simulink model "iiwa_v_1"  (R2015a)
settings: Solver=ode3  StartTime=0.0  StopTime=10  FixedStep=0.001  RelTol=1e-3
undefined symbols (not defined in the file or in its folder): X, Y, Z
libraries: sm_lib x40, nesl_utility x22
settings Model: Creator=alaa.alassi1  LastModifiedBy=robotic

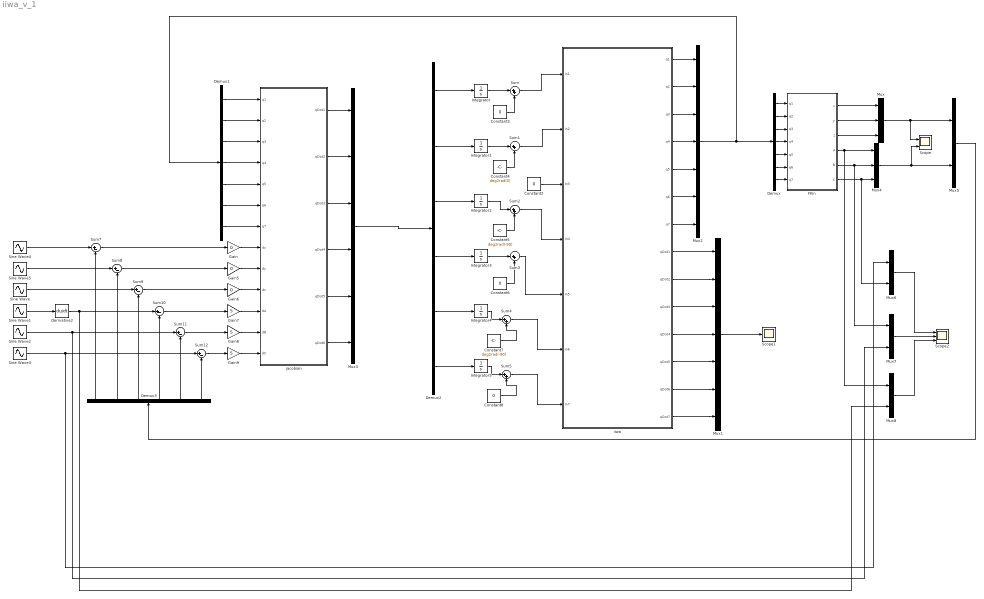
== system iiwa_v_1 ==
  Constant{2..3,6,8} (4 alike) : Constant  Value=0
  Constant4 : Constant  Value=deg2rad(0)
  Constant5 : Constant  Value=deg2rad(-90)
  Constant7 : Constant  Value=deg2rad(-90)
  Demux : Demux  Outputs=7
  Demux1 : Demux  Outputs=7
  Demux2 : Demux  Outputs=6
  Demux3 : Demux  Outputs=6
  Derivative2 : Derivative
  FKin : MATLAB Function  TreatAsAtomicUnit=on
  Gain : Gain  Gain=0
  Gain5 : Gain  Gain=0
  Gain6 : Gain  Gain=0
  Gain7 : Gain  Gain=5
  Gain8 : Gain  Gain=5
  Gain9 : Gain  Gain=5
  Integrator{,1..5} (6 alike) : Integrator
  Mux : Mux  Inputs=3
  Mux1 : Mux  Inputs=7
  Mux2 : Mux  Inputs=7
  Mux3 : Mux  Inputs=6
  Mux4 : Mux  Inputs=3
  Mux{5..8} (4 alike) : Mux  Inputs=2
  Scope : Scope  NumInputPorts=2
      settings: YMin=-5~-5  YMax=5~5
  Scope1 : Scope
  Scope2 : Scope  NumInputPorts=3
      settings: YMin=-5~-5~-5  YMax=5~5~5  SaveName=ScopeData2
  Sine Wave : Sin  Amplitude=0.1  Bias=0.7067  Frequency=4  SampleTime=0
  Sine Wave1 : Sin  SampleTime=0
  Sine Wave2 : Sin  SampleTime=0
  Sine Wave3 : Sin  SampleTime=0
  Sine Wave4 : Sin  Amplitude=0.1  Bias=0.7067  Frequency=4  SampleTime=0
  Sine Wave5 : Sin  Amplitude=0.1  Bias=0.7067  Frequency=4  SampleTime=0
  Sum{,1..5} (6 alike) : Sum  Inputs=|++
  Sum{7..12} (6 alike) : Sum  Inputs=|+-
  iiwa : Subsystem
  jacobian : MATLAB Function  TreatAsAtomicUnit=on
  wires:
  FKin/1(x) -> Mux/1
  FKin/2(y) -> Mux/2
  FKin/3(z) -> Mux/3
  Mux/1 -> Scope/1, Mux5/1
  Mux1/1 -> Scope1/1
  iiwa/8(qDot1) -> Mux1/1
  iiwa/9(qDot2) -> Mux1/2
  iiwa/10(qDot3) -> Mux1/3
  iiwa/11(qDot4) -> Mux1/4
  iiwa/12(qDot5) -> Mux1/5
  iiwa/13(qDot6) -> Mux1/6
  iiwa/14(qDot7) -> Mux1/7
  iiwa/1(q1) -> Mux2/1
  iiwa/3(q3) -> Mux2/3
  iiwa/4(q4) -> Mux2/4
  iiwa/5(q5) -> Mux2/5
  iiwa/6(q6) -> Mux2/6
  iiwa/7(q7) -> Mux2/7
  Demux/1 -> FKin/1(q1)
  Demux/2 -> FKin/2(q2)
  Demux/3 -> FKin/3(q3)
  Demux/4 -> FKin/4(q4)
  Demux/5 -> FKin/5(q5)
  Demux/6 -> FKin/6(q6)
  Demux/7 -> FKin/7(q7)
  Demux1/1 -> jacobian/1(q1)
  Demux1/2 -> jacobian/2(q2)
  Demux1/3 -> jacobian/3(q3)
  Demux1/4 -> jacobian/4(q4)
  Demux1/5 -> jacobian/5(q5)
  Demux1/6 -> jacobian/6(q6)
  Demux1/7 -> jacobian/7(q7)
  Mux2/1 -> Demux1/1, Demux/1
  jacobian/1(qDot1) -> Mux3/1
  jacobian/2(qDot2) -> Mux3/2
  jacobian/3(qDot3) -> Mux3/3
  jacobian/4(qDot4) -> Mux3/4
  jacobian/5(qDot5) -> Mux3/5
  jacobian/6(qDot6) -> Mux3/6
  Constant2/1 -> iiwa/3(In3)
  Demux2/1 -> Integrator/1
  Demux2/2 -> Integrator1/1
  Demux2/3 -> Integrator2/1
  Demux2/4 -> Integrator3/1
  Demux2/5 -> Integrator4/1
  Demux2/6 -> Integrator5/1
  Integrator/1 -> Sum/1
  Sum/1 -> iiwa/1(In1)
  Constant3/1 -> Sum/2
  Integrator1/1 -> Sum1/1
  Sum1/1 -> iiwa/2(In2)
  Constant4/1 -> Sum1/2
  Integrator2/1 -> Sum2/1
  Sum2/1 -> iiwa/4(In4)
  Constant5/1 -> Sum2/2
  Integrator3/1 -> Sum3/1
  Sum3/1 -> iiwa/5(In5)
  Constant6/1 -> Sum3/2
  Integrator4/1 -> Sum4/1
  Sum4/1 -> iiwa/6(In6)
  Constant7/1 -> Sum4/2
  Integrator5/1 -> Sum5/1
  Sum5/1 -> iiwa/7(In7)
  Constant8/1 -> Sum5/2
  Mux3/1 -> Demux2/1
  iiwa/2(q2) -> Mux2/2
  FKin/4(A) -> Mux8/1, Mux4/1
  FKin/5(B) -> Mux7/1, Mux4/2
  FKin/6(C) -> Mux6/2, Mux4/3
  Mux4/1 -> Scope/2, Mux5/2
  Gain/1 -> jacobian/8(dx)
  Gain5/1 -> jacobian/9(dy)
  Gain6/1 -> jacobian/10(dz)
  Gain7/1 -> jacobian/11(dA)
  Gain8/1 -> jacobian/12(dB)
  Gain9/1 -> jacobian/13(dC)
  Sum7/1 -> Gain/1
  Sum8/1 -> Gain5/1
  Sum9/1 -> Gain6/1
  Sum10/1 -> Gain7/1
  Sum11/1 -> Gain8/1
  Sum12/1 -> Gain9/1
  Mux5/1 -> Demux3/1
  Demux3/6 -> Sum12/2
  Demux3/1 -> Sum7/2
  Demux3/2 -> Sum8/2
  Demux3/3 -> Sum9/2
  Demux3/4 -> Sum10/2
  Demux3/5 -> Sum11/2
  Sine Wave/1 -> Sum9/1
  Sine Wave4/1 -> Sum7/1
  Sine Wave5/1 -> Sum8/1
  Mux6/1 -> Scope2/1
  Sine Wave2/1 -> Mux7/2, Sum11/1
  Sine Wave1/1 -> Derivative2/1
  Mux7/1 -> Scope2/2
  Mux8/1 -> Scope2/3
  Derivative2/1 -> Sum10/1, Mux8/2
  Sine Wave3/1 -> Sum12/1, Mux6/1

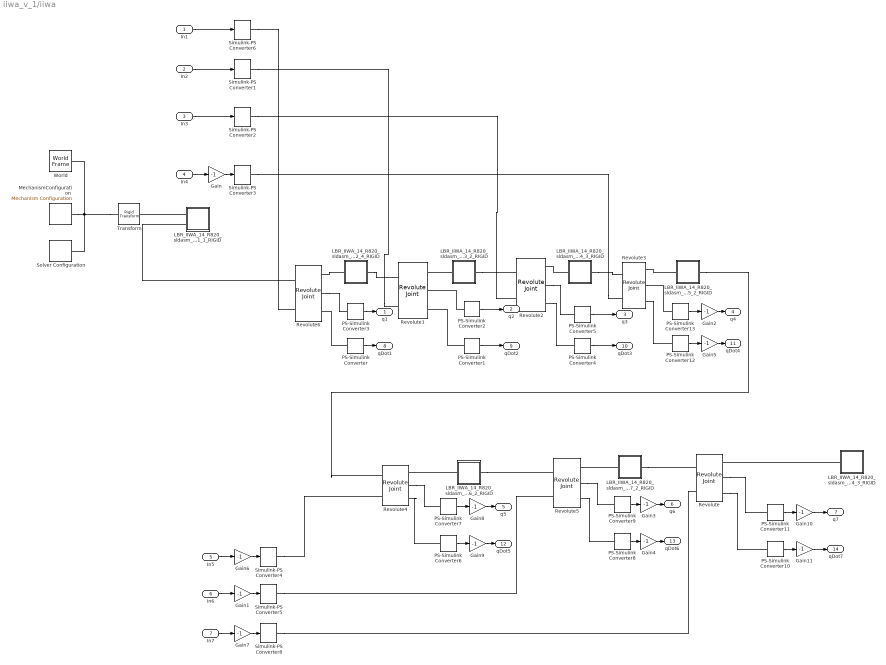
== system iiwa_v_1/iiwa ==
  In1 : Inport
  In2 : Inport  Port=2
  In3 : Inport  Port=3
  In4 : Inport  Port=4
  In5 : Inport  Port=5
  In6 : Inport  Port=6
  In7 : Inport  Port=7
  Gain{,1..11} (12 alike) : Gain  Gain=-1
  LBR_IIWA_14_R820_sldasm_Part_14_3_RIGID : Subsystem
  LBR_IIWA_14_R820_sldasm_Part_1_1_RIGID : Subsystem
  LBR_IIWA_14_R820_sldasm_Part_2_4_RIGID : Subsystem
  LBR_IIWA_14_R820_sldasm_Part_3_2_RIGID : Subsystem
  LBR_IIWA_14_R820_sldasm_Part_4_3_RIGID : Subsystem
  LBR_IIWA_14_R820_sldasm_Part_5_2_RIGID : Subsystem
  LBR_IIWA_14_R820_sldasm_Part_6_2_RIGID : Subsystem
  LBR_IIWA_14_R820_sldasm_Part_7_2_RIGID : Subsystem
  MechanismConfiguration : sm_lib/Utilities/Mechanism Configuration  UniformGravity=Constant  GravityVector=[0 -0 -0]  GravityUnits=m/s^2  LinearizationDelta=0.001  BlockFunction=simmechanics.library.utilities.mechanism_configuration
  PS-Simulink Converter{,1..13} (14 alike) : nesl_utility/PS-Simulink Converter  PhysicalDomain=network_engine_domain  SubClassName=ps_output  LeftPortType=input  RightPortType=output  PseudoPeriodic=off  Frequencies=[]  Unit=1  AffineConversion=off
  Revolute : sm_lib/Joints/Revolute Joint  SenseConstraintForce=off  SenseConstraintForceX=off  SenseConstraintForceY=off  SenseConstraintForceZ=off  SenseConstraintTorque=off  SenseConstraintTorqueX=off  SenseConstraintTorqueY=off  SenseConstraintTorqueZ=off  SenseTotalForce=off  SenseTotalForceX=off  SenseTotalForceY=off  SenseTotalForceZ=off  SenseTotalTorque=off  SenseTotalTorqueX=off  SenseTotalTorqueY=off  SenseTotalTorqueZ=off  CompositeWrenchDir=FollowerOnBase  CompositeWrenchFrame=BaseFrame  EquilibriumPosition=0  EquilibriumPositionUnits=rad  SpringStiffness=0  SpringStiffnessUnits=m*N/rad  DampingCoefficient=0  DampingCoefficientUnits=m*s*N/rad  TorqueActuationMode=ComputedTorque  MotionActuationMode=InputMotion  SensePosition=on  SenseVelocity=on  SenseAcceleration=off  SenseTorqueForce=off  PositionTargetSpecify=off  PositionTargetPriority=Low  PositionTargetValue=0  PositionTargetValueUnits=deg  VelocityTargetSpecify=off  VelocityTargetPriority=High  VelocityTargetValue=0  VelocityTargetValueUnits=deg/s  BlockFunction=simmechanics.library.joints.revolute_joint
  Revolute1 : sm_lib/Joints/Revolute Joint  SenseConstraintForce=off  SenseConstraintForceX=off  SenseConstraintForceY=off  SenseConstraintForceZ=off  SenseConstraintTorque=off  SenseConstraintTorqueX=off  SenseConstraintTorqueY=off  SenseConstraintTorqueZ=off  SenseTotalForce=off  SenseTotalForceX=off  SenseTotalForceY=off  SenseTotalForceZ=off  SenseTotalTorque=off  SenseTotalTorqueX=off  SenseTotalTorqueY=off  SenseTotalTorqueZ=off  CompositeWrenchDir=FollowerOnBase  CompositeWrenchFrame=BaseFrame  EquilibriumPosition=0  EquilibriumPositionUnits=rad  SpringStiffness=0  SpringStiffnessUnits=m*N/rad  DampingCoefficient=0  DampingCoefficientUnits=m*s*N/rad  TorqueActuationMode=ComputedTorque  MotionActuationMode=InputMotion  SensePosition=on  SenseVelocity=on  SenseAcceleration=off  SenseTorqueForce=off  PositionTargetSpecify=on  PositionTargetPriority=Low  PositionTargetValue=0  PositionTargetValueUnits=deg  VelocityTargetSpecify=off  VelocityTargetPriority=Low  VelocityTargetValue=0  VelocityTargetValueUnits=deg/s  BlockFunction=simmechanics.library.joints.revolute_joint
  Revolute2 : sm_lib/Joints/Revolute Joint  SenseConstraintForce=off  SenseConstraintForceX=off  SenseConstraintForceY=off  SenseConstraintForceZ=off  SenseConstraintTorque=off  SenseConstraintTorqueX=off  SenseConstraintTorqueY=off  SenseConstraintTorqueZ=off  SenseTotalForce=off  SenseTotalForceX=off  SenseTotalForceY=off  SenseTotalForceZ=off  SenseTotalTorque=off  SenseTotalTorqueX=off  SenseTotalTorqueY=off  SenseTotalTorqueZ=off  CompositeWrenchDir=FollowerOnBase  CompositeWrenchFrame=BaseFrame  EquilibriumPosition=0  EquilibriumPositionUnits=rad  SpringStiffness=0  SpringStiffnessUnits=m*N/rad  DampingCoefficient=0  DampingCoefficientUnits=m*s*N/rad  TorqueActuationMode=ComputedTorque  MotionActuationMode=InputMotion  SensePosition=on  SenseVelocity=on  SenseAcceleration=off  SenseTorqueForce=off  PositionTargetSpecify=off  PositionTargetPriority=Low  PositionTargetValue=0  PositionTargetValueUnits=deg  VelocityTargetSpecify=off  VelocityTargetPriority=High  VelocityTargetValue=0  VelocityTargetValueUnits=deg/s  BlockFunction=simmechanics.library.joints.revolute_joint
  Revolute3 : sm_lib/Joints/Revolute Joint  SenseConstraintForce=off  SenseConstraintForceX=off  SenseConstraintForceY=off  SenseConstraintForceZ=off  SenseConstraintTorque=off  SenseConstraintTorqueX=off  SenseConstraintTorqueY=off  SenseConstraintTorqueZ=off  SenseTotalForce=off  SenseTotalForceX=off  SenseTotalForceY=off  SenseTotalForceZ=off  SenseTotalTorque=off  SenseTotalTorqueX=off  SenseTotalTorqueY=off  SenseTotalTorqueZ=off  CompositeWrenchDir=FollowerOnBase  CompositeWrenchFrame=BaseFrame  EquilibriumPosition=0  EquilibriumPositionUnits=rad  SpringStiffness=0  SpringStiffnessUnits=m*N/rad  DampingCoefficient=0  DampingCoefficientUnits=m*s*N/rad  TorqueActuationMode=ComputedTorque  MotionActuationMode=InputMotion  SensePosition=on  SenseVelocity=on  SenseAcceleration=off  SenseTorqueForce=off  PositionTargetSpecify=off  PositionTargetPriority=Low  PositionTargetValue=60  PositionTargetValueUnits=deg  VelocityTargetSpecify=off  VelocityTargetPriority=High  VelocityTargetValue=0  VelocityTargetValueUnits=deg/s  BlockFunction=simmechanics.library.joints.revolute_joint
  Revolute4 : sm_lib/Joints/Revolute Joint  SenseConstraintForce=off  SenseConstraintForceX=off  SenseConstraintForceY=off  SenseConstraintForceZ=off  SenseConstraintTorque=off  SenseConstraintTorqueX=off  SenseConstraintTorqueY=off  SenseConstraintTorqueZ=off  SenseTotalForce=off  SenseTotalForceX=off  SenseTotalForceY=off  SenseTotalForceZ=off  SenseTotalTorque=off  SenseTotalTorqueX=off  SenseTotalTorqueY=off  SenseTotalTorqueZ=off  CompositeWrenchDir=FollowerOnBase  CompositeWrenchFrame=BaseFrame  EquilibriumPosition=0  EquilibriumPositionUnits=rad  SpringStiffness=0  SpringStiffnessUnits=m*N/rad  DampingCoefficient=0  DampingCoefficientUnits=m*s*N/rad  TorqueActuationMode=ComputedTorque  MotionActuationMode=InputMotion  SensePosition=on  SenseVelocity=on  SenseAcceleration=off  SenseTorqueForce=off  PositionTargetSpecify=off  PositionTargetPriority=Low  PositionTargetValue=0  PositionTargetValueUnits=deg  VelocityTargetSpecify=off  VelocityTargetPriority=High  VelocityTargetValue=0  VelocityTargetValueUnits=deg/s  BlockFunction=simmechanics.library.joints.revolute_joint
  Revolute5 : sm_lib/Joints/Revolute Joint  SenseConstraintForce=off  SenseConstraintForceX=off  SenseConstraintForceY=off  SenseConstraintForceZ=off  SenseConstraintTorque=off  SenseConstraintTorqueX=off  SenseConstraintTorqueY=off  SenseConstraintTorqueZ=off  SenseTotalForce=off  SenseTotalForceX=off  SenseTotalForceY=off  SenseTotalForceZ=off  SenseTotalTorque=off  SenseTotalTorqueX=off  SenseTotalTorqueY=off  SenseTotalTorqueZ=off  CompositeWrenchDir=FollowerOnBase  CompositeWrenchFrame=BaseFrame  EquilibriumPosition=0  EquilibriumPositionUnits=rad  SpringStiffness=0  SpringStiffnessUnits=m*N/rad  DampingCoefficient=0  DampingCoefficientUnits=m*s*N/rad  TorqueActuationMode=ComputedTorque  MotionActuationMode=InputMotion  SensePosition=on  SenseVelocity=on  SenseAcceleration=off  SenseTorqueForce=off  PositionTargetSpecify=off  PositionTargetPriority=Low  PositionTargetValue=-90  PositionTargetValueUnits=deg  VelocityTargetSpecify=off  VelocityTargetPriority=High  VelocityTargetValue=0  VelocityTargetValueUnits=deg/s  BlockFunction=simmechanics.library.joints.revolute_joint
  Revolute6 : sm_lib/Joints/Revolute Joint  SenseConstraintForce=off  SenseConstraintForceX=off  SenseConstraintForceY=off  SenseConstraintForceZ=off  SenseConstraintTorque=off  SenseConstraintTorqueX=off  SenseConstraintTorqueY=off  SenseConstraintTorqueZ=off  SenseTotalForce=off  SenseTotalForceX=off  SenseTotalForceY=off  SenseTotalForceZ=off  SenseTotalTorque=off  SenseTotalTorqueX=off  SenseTotalTorqueY=off  SenseTotalTorqueZ=off  CompositeWrenchDir=FollowerOnBase  CompositeWrenchFrame=BaseFrame  EquilibriumPosition=0  EquilibriumPositionUnits=rad  SpringStiffness=0  SpringStiffnessUnits=m*N/rad  DampingCoefficient=0  DampingCoefficientUnits=m*s*N/rad  TorqueActuationMode=ComputedTorque  MotionActuationMode=InputMotion  SensePosition=on  SenseVelocity=on  SenseAcceleration=off  SenseTorqueForce=off  PositionTargetSpecify=off  PositionTargetPriority=Low  PositionTargetValue=0  PositionTargetValueUnits=deg  VelocityTargetSpecify=off  VelocityTargetPriority=High  VelocityTargetValue=1  VelocityTargetValueUnits=rad/s  BlockFunction=simmechanics.library.joints.revolute_joint
  Simulink-PS Converter{1..5,8} (6 alike) : nesl_utility/Simulink-PS Converter  PhysicalDomain=network_engine_domain  SubClassName=ps_input  LeftPortType=input  RightPortType=output  PseudoPeriodic=off  Frequencies=[]  NoiseDistribution=none  NoiseParameters=[]  Unit=rad  AffineConversion=on  InputFiltering=on  SimscapeFilterOrder=2  InputFilterTimeConstant=0.001  UdotUserProvided=1
  Simulink-PS Converter6 : nesl_utility/Simulink-PS Converter  PhysicalDomain=network_engine_domain  SubClassName=ps_input  LeftPortType=input  RightPortType=output  PseudoPeriodic=off  Frequencies=[]  NoiseDistribution=none  NoiseParameters=[]  Unit=rad  AffineConversion=on  InputFiltering=on  SimscapeFilterOrder=2  InputFilterTimeConstant=0.001  UdotUserProvided=2
  Solver Configuration : nesl_utility/Solver Configuration  PhysicalDomain=network_engine_domain  SubClassName=solver  LeftPortType=input  RightPortType=generic  Accelerate=off  Tones=[]  Harmonics=[]  SimulateNoise=off  Profile=off  UseLocalSampling=off  EnableSwitchedLinearOptims=on  FrequencyDomain=off  UseCCode=off  RelTol=0.001  AbsTol=1e-06  MinStep=1e-09  ToWorkspace=off  RevertToSquareIcSolve=off  NumHomotopyIterations=100  DoDC=off  ResidualTolerance=1e-09  UseLocalSolver=off  LocalSolverChoice=NE_BACKWARD_EULER_ADVANCER  LocalSolverSampleTime=0.001  DoFixedCost=off  MaxNonlinIter=3  MaxModeIter=2  LinearAlgebra=Sparse  DelaysMemoryBudget=1024  AutomaticFiltering=on  FilteringTimeConstant=0.001
  Transform : sm_lib/Frames and Transforms/Rigid Transform  TranslationMethod=Cartesian  TranslationLengthUnit=mm  TranslationStandardAxis=+Z  TranslationStandardOffset=0  TranslationCartesianOffset=[119.17615287075404 -10.082715490568717 -56.037583436526596]  TranslationROffset=0  TranslationROffsetUnits=m  TranslationZOffset=0  TranslationZOffsetUnits=m  TranslationThetaOffset=0  TranslationThetaOffsetUnits=deg  RotationMethod=None  RotationAngleUnits=deg  RotationStandardAxis=+Z  RotationAngle=0.0  RotationArbitraryAxis=[0 0 1]  FollAlignAxisA=+X  BaseAlignAxisA=+Y  FollAlignAxisB=+Y  BaseAlignAxisB=+Z  RotationMatrix=[1 0 0; 0 1 0; 0 0 1]  BlockFunction=simmechanics.library.frames_transforms.rigid_transform
  World : sm_lib/Frames and Transforms/World Frame  BlockFunction=simmechanics.library.frames_transforms.world_frame
  q1 : Outport
  q2 : Outport  Port=2
  q3 : Outport  Port=3
  q4 : Outport  Port=4
  q5 : Outport  Port=5
  q6 : Outport  Port=6
  q7 : Outport  Port=7
  qDot1 : Outport  Port=8
  qDot2 : Outport  Port=9
  qDot3 : Outport  Port=10
  qDot4 : Outport  Port=11
  qDot5 : Outport  Port=12
  qDot6 : Outport  Port=13
  qDot7 : Outport  Port=14
  wires:
  PS-Simulink Converter12/1 -> Gain5/1
  PS-Simulink Converter13/1 -> Gain2/1
  In3/1 -> Simulink-PS Converter2/1
  In6/1 -> Gain1/1
  PS-Simulink Converter11/1 -> Gain10/1
  In1/1 -> Simulink-PS Converter6/1
  In2/1 -> Simulink-PS Converter1/1
  PS-Simulink Converter5/1 -> q3/1
  PS-Simulink Converter1/1 -> qDot2/1
  PS-Simulink Converter4/1 -> qDot3/1
  PS-Simulink Converter6/1 -> Gain9/1
  PS-Simulink Converter2/1 -> q2/1
  PS-Simulink Converter3/1 -> q1/1
  PS-Simulink Converter/1 -> qDot1/1
  Gain/1 -> Simulink-PS Converter3/1
  In4/1 -> Gain/1
  Gain1/1 -> Simulink-PS Converter5/1
  Gain2/1 -> q4/1
  PS-Simulink Converter9/1 -> Gain3/1
  Gain3/1 -> q6/1
  PS-Simulink Converter8/1 -> Gain4/1
  Gain4/1 -> qDot6/1
  Gain5/1 -> qDot4/1
  In5/1 -> Gain6/1
  Gain6/1 -> Simulink-PS Converter4/1
  Gain7/1 -> Simulink-PS Converter8/1
  In7/1 -> Gain7/1
  PS-Simulink Converter7/1 -> Gain8/1
  Gain8/1 -> q5/1
  Gain9/1 -> qDot5/1
  Gain10/1 -> q7/1
  PS-Simulink Converter10/1 -> Gain11/1
  Gain11/1 -> qDot7/1
  connections:
  LBR_IIWA_14_R820_sldasm_Part_2_4_RIGID/RConn1 -- Revolute1/LConn1
  LBR_IIWA_14_R820_sldasm_Part_14_3_RIGID/LConn1 -- Revolute/RConn1
  LBR_IIWA_14_R820_sldasm_Part_3_2_RIGID/RConn1 -- Revolute2/LConn1
  LBR_IIWA_14_R820_sldasm_Part_4_3_RIGID/LConn1 -- Revolute2/RConn1
  LBR_IIWA_14_R820_sldasm_Part_3_2_RIGID/LConn1 -- Revolute1/RConn1
  Transform/LConn1 -- World/RConn1 -- Solver Configuration/RConn1 -- MechanismConfiguration/RConn1
  LBR_IIWA_14_R820_sldasm_Part_6_2_RIGID/RConn1 -- Revolute5/LConn1
  LBR_IIWA_14_R820_sldasm_Part_5_2_RIGID/RConn1 -- Revolute4/LConn1
  LBR_IIWA_14_R820_sldasm_Part_7_2_RIGID/LConn1 -- Revolute5/RConn1
  LBR_IIWA_14_R820_sldasm_Part_1_1_RIGID/LConn1 -- Transform/RConn1
  LBR_IIWA_14_R820_sldasm_Part_7_2_RIGID/RConn1 -- Revolute/LConn1
  LBR_IIWA_14_R820_sldasm_Part_6_2_RIGID/LConn1 -- Revolute4/RConn1
  Revolute3/RConn3 -- PS-Simulink Converter12/LConn1
  PS-Simulink Converter1/LConn1 -- Revolute1/RConn3
  PS-Simulink Converter13/LConn1 -- Revolute3/RConn2
  PS-Simulink Converter/LConn1 -- Revolute6/RConn3
  Revolute6/RConn2 -- PS-Simulink Converter3/LConn1
  Simulink-PS Converter1/RConn1 -- Revolute1/LConn2
  LBR_IIWA_14_R820_sldasm_Part_4_3_RIGID/RConn1 -- Revolute3/LConn1
  LBR_IIWA_14_R820_sldasm_Part_5_2_RIGID/LConn1 -- Revolute3/RConn1
  LBR_IIWA_14_R820_sldasm_Part_1_1_RIGID/LConn2 -- Revolute6/LConn1
  Revolute6/RConn1 -- LBR_IIWA_14_R820_sldasm_Part_2_4_RIGID/LConn1
  Simulink-PS Converter2/RConn1 -- Revolute2/LConn2
  Simulink-PS Converter3/RConn1 -- Revolute3/LConn2
  Simulink-PS Converter4/RConn1 -- Revolute4/LConn2
  Simulink-PS Converter5/RConn1 -- Revolute5/LConn2
  Simulink-PS Converter8/RConn1 -- Revolute/LConn2
  Revolute/RConn2 -- PS-Simulink Converter11/LConn1
  PS-Simulink Converter2/LConn1 -- Revolute1/RConn2
  Revolute/RConn3 -- PS-Simulink Converter10/LConn1
  Simulink-PS Converter6/RConn1 -- Revolute6/LConn2
  Revolute2/RConn3 -- PS-Simulink Converter4/LConn1
  Revolute4/RConn2 -- PS-Simulink Converter7/LConn1
  Revolute5/RConn3 -- PS-Simulink Converter8/LConn1
  Revolute2/RConn2 -- PS-Simulink Converter5/LConn1
  Revolute4/RConn3 -- PS-Simulink Converter6/LConn1
  Revolute5/RConn2 -- PS-Simulink Converter9/LConn1

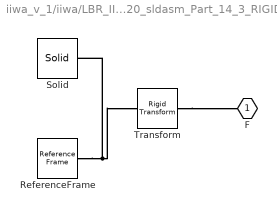
== system iiwa_v_1/iiwa/LBR_IIWA_14_R820_sldasm_Part_14_3_RIGID ==
  ReferenceFrame : sm_lib/Frames and Transforms/Reference Frame  BlockFunction=simmechanics.library.frames_transforms.reference_frame
  Solid : sm_lib/Body Elements/Solid  InertiaType=Custom  Mass=0.31121894529121702  MassUnits=kg  CenterOfMass=[0.014528621653147699 0.087032798846967588 1278.3655137735861]  CenterOfMassUnits=mm  MomentsOfInertia=[222.42389382502736 221.16881041551065 342.04081748406088]  MomentsOfInertiaUnits=kg*mm^2  ProductsOfInertia=[-0.22311621312267468 -0.062033496808603497 0.11472620552029689]  ProductsOfInertiaUnits=kg*mm^2  DensityBased=on  Density=1000  DensityUnits=kg/(m^3)  GraphicType=FromGeometry  MarkerShape=Sphere  MarkerSize=10  MarkerSizeUnits=m  GraphicVisPropType=SimpleVisualProperties  GraphicDiffuseColor=[0.40000000000000002 0.40000000000000002 0.40000000000000002]  GraphicSpecularColor=[0.5 0.5 0.5 1.0]  GraphicAmbientColor=[0.15 0.15 0.15 1.0]  GraphicEmissiveColor=[0.0 0.0 0.0 1.0]  GraphicShininess=75  GraphicOpacity=1  GeometryShape=FromFile  RectangleSize=[1 1]  RectangleSizeUnits=m  BrickDimensions=[1 1 1]  BrickDimensionUnits=m  CylinderRadius=1  CylinderRadiusUnits=m  CylinderLength=1  CylinderLengthUnits=m  SphereRadius=1  SphereRadiusUnits=m  EllipsoidRadii=[1 1 1]  EllipsoidRadiiUnits=m  ExtrusionCrossSection=[1 1; -1 1; -1 -1; 1 -1]  ExtrusionCrossSectionUnits=m  ExtrusionLength=1  ExtrusionLengthUnits=m  PolygonNumSides=3  PolygonOuterRadius=1  PolygonOuterRadiusUnits=m  ExtGeomFileType=STL  ExtGeomFileName=LBR IIWA 14 R820.sldasm-Part-14_Default_sldprt.STL  ExtGeomFileUnits=mm  RevolutionCrossSection=[1 1; 1 -1; 2 -1; 2 1]  RevolutionCrossSectionUnits=m  RevolutionExtent=Full  RevolutionAngle=180  RevolutionAngleUnits=deg  BlockFunction=simmechanics.library.body_elements.solid
  Transform : sm_lib/Frames and Transforms/Rigid Transform  TranslationMethod=Cartesian  TranslationLengthUnit=mm  TranslationStandardAxis=+Z  TranslationStandardOffset=0  TranslationCartesianOffset=[1.4210854715202004e-14 0 1260.9522642316304]  TranslationROffset=0  TranslationROffsetUnits=m  TranslationZOffset=0  TranslationZOffsetUnits=m  TranslationThetaOffset=0  TranslationThetaOffsetUnits=deg  RotationMethod=ArbitraryAxis  RotationAngleUnits=rad  RotationStandardAxis=+Z  RotationAngle=3.1415926535897931  RotationArbitraryAxis=[1 0 0]  FollAlignAxisA=+X  BaseAlignAxisA=+Y  FollAlignAxisB=+Y  BaseAlignAxisB=+Z  RotationMatrix=[1 0 0; 0 1 0; 0 0 1]  BlockFunction=simmechanics.library.frames_transforms.rigid_transform
  F : PMIOPort  Port=1  Side=Left
  connections:
  Solid/RConn1 -- ReferenceFrame/RConn1 -- Transform/LConn1
  Transform/RConn1 -- F/RConn1

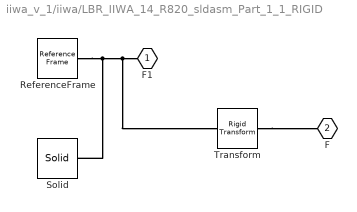
== system iiwa_v_1/iiwa/LBR_IIWA_14_R820_sldasm_Part_1_1_RIGID ==
  ReferenceFrame : sm_lib/Frames and Transforms/Reference Frame  BlockFunction=simmechanics.library.frames_transforms.reference_frame
  Solid : sm_lib/Body Elements/Solid  InertiaType=Custom  Mass=5.4763191824074191  MassUnits=kg  CenterOfMass=[-12.821238335721649 -9.0947303464757157e-05 71.506762335264654]  CenterOfMassUnits=mm  MomentsOfInertia=[24255.461347568311 30834.856026538371 33479.935107594152]  MomentsOfInertiaUnits=kg*mm^2  ProductsOfInertia=[-0.013206934110401594 676.36516175109693 0.22783758420025393]  ProductsOfInertiaUnits=kg*mm^2  DensityBased=on  Density=1000  DensityUnits=kg/(m^3)  GraphicType=FromGeometry  MarkerShape=Sphere  MarkerSize=10  MarkerSizeUnits=m  GraphicVisPropType=SimpleVisualProperties  GraphicDiffuseColor=[0.40000000000000002 0.40000000000000002 0.40000000000000002]  GraphicSpecularColor=[0.5 0.5 0.5 1.0]  GraphicAmbientColor=[0.15 0.15 0.15 1.0]  GraphicEmissiveColor=[0.0 0.0 0.0 1.0]  GraphicShininess=75  GraphicOpacity=1  GeometryShape=FromFile  RectangleSize=[1 1]  RectangleSizeUnits=m  BrickDimensions=[1 1 1]  BrickDimensionUnits=m  CylinderRadius=1  CylinderRadiusUnits=m  CylinderLength=1  CylinderLengthUnits=m  SphereRadius=1  SphereRadiusUnits=m  EllipsoidRadii=[1 1 1]  EllipsoidRadiiUnits=m  ExtrusionCrossSection=[1 1; -1 1; -1 -1; 1 -1]  ExtrusionCrossSectionUnits=m  ExtrusionLength=1  ExtrusionLengthUnits=m  PolygonNumSides=3  PolygonOuterRadius=1  PolygonOuterRadiusUnits=m  ExtGeomFileType=STL  ExtGeomFileName=LBR IIWA 14 R820.sldasm-Part-1_Default_sldprt.STL  ExtGeomFileUnits=mm  RevolutionCrossSection=[1 1; 1 -1; 2 -1; 2 1]  RevolutionCrossSectionUnits=m  RevolutionExtent=Full  RevolutionAngle=180  RevolutionAngleUnits=deg  BlockFunction=simmechanics.library.body_elements.solid
  Transform : sm_lib/Frames and Transforms/Rigid Transform  TranslationMethod=Cartesian  TranslationLengthUnit=mm  TranslationStandardAxis=+Z  TranslationStandardOffset=0  TranslationCartesianOffset=[0 0 0]  TranslationROffset=0  TranslationROffsetUnits=m  TranslationZOffset=0  TranslationZOffsetUnits=m  TranslationThetaOffset=0  TranslationThetaOffsetUnits=deg  RotationMethod=ArbitraryAxis  RotationAngleUnits=rad  RotationStandardAxis=+Z  RotationAngle=0  RotationArbitraryAxis=[0 0 0]  FollAlignAxisA=+X  BaseAlignAxisA=+Y  FollAlignAxisB=+Y  BaseAlignAxisB=+Z  RotationMatrix=[1 0 0; 0 1 0; 0 0 1]  BlockFunction=simmechanics.library.frames_transforms.rigid_transform
  F1 : PMIOPort  Port=1  Side=Left
  F : PMIOPort  Port=2  Side=Left
  connections:
  Solid/RConn1 -- ReferenceFrame/RConn1 -- Transform/LConn1 -- F1/RConn1
  Transform/RConn1 -- F/RConn1

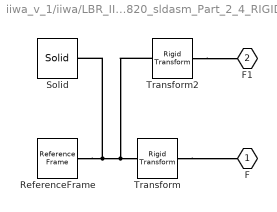
== system iiwa_v_1/iiwa/LBR_IIWA_14_R820_sldasm_Part_2_4_RIGID ==
  ReferenceFrame : sm_lib/Frames and Transforms/Reference Frame  BlockFunction=simmechanics.library.frames_transforms.reference_frame
  Solid : sm_lib/Body Elements/Solid  InertiaType=Custom  Mass=4.1083201278586756  MassUnits=kg  CenterOfMass=[0.002023674017061809 -33.791806722636508 279.89622818117567]  CenterOfMassUnits=mm  MomentsOfInertia=[32979.16478681071 33271.017005185153 12325.355527303365]  MomentsOfInertiaUnits=kg*mm^2  ProductsOfInertia=[4923.2398738864858 -0.93636485022231042 0.93559130304616511]  ProductsOfInertiaUnits=kg*mm^2  DensityBased=on  Density=1000  DensityUnits=kg/(m^3)  GraphicType=FromGeometry  MarkerShape=Sphere  MarkerSize=10  MarkerSizeUnits=m  GraphicVisPropType=SimpleVisualProperties  GraphicDiffuseColor=[1 0.40000000000000002 0]  GraphicSpecularColor=[0.5 0.5 0.5 1.0]  GraphicAmbientColor=[0.15 0.15 0.15 1.0]  GraphicEmissiveColor=[0.0 0.0 0.0 1.0]  GraphicShininess=75  GraphicOpacity=1  GeometryShape=FromFile  RectangleSize=[1 1]  RectangleSizeUnits=m  BrickDimensions=[1 1 1]  BrickDimensionUnits=m  CylinderRadius=1  CylinderRadiusUnits=m  CylinderLength=1  CylinderLengthUnits=m  SphereRadius=1  SphereRadiusUnits=m  EllipsoidRadii=[1 1 1]  EllipsoidRadiiUnits=m  ExtrusionCrossSection=[1 1; -1 1; -1 -1; 1 -1]  ExtrusionCrossSectionUnits=m  ExtrusionLength=1  ExtrusionLengthUnits=m  PolygonNumSides=3  PolygonOuterRadius=1  PolygonOuterRadiusUnits=m  ExtGeomFileType=STL  ExtGeomFileName=LBR IIWA 14 R820.sldasm-Part-2_Default_sldprt.STL  ExtGeomFileUnits=mm  RevolutionCrossSection=[1 1; 1 -1; 2 -1; 2 1]  RevolutionCrossSectionUnits=m  RevolutionExtent=Full  RevolutionAngle=180  RevolutionAngleUnits=deg  BlockFunction=simmechanics.library.body_elements.solid
  Transform : sm_lib/Frames and Transforms/Rigid Transform  TranslationMethod=Cartesian  TranslationLengthUnit=mm  TranslationStandardAxis=+Z  TranslationStandardOffset=0  TranslationCartesianOffset=[0 0 0]  TranslationROffset=0  TranslationROffsetUnits=m  TranslationZOffset=0  TranslationZOffsetUnits=m  TranslationThetaOffset=0  TranslationThetaOffsetUnits=deg  RotationMethod=ArbitraryAxis  RotationAngleUnits=rad  RotationStandardAxis=+Z  RotationAngle=0  RotationArbitraryAxis=[0 0 0]  FollAlignAxisA=+X  BaseAlignAxisA=+Y  FollAlignAxisB=+Y  BaseAlignAxisB=+Z  RotationMatrix=[1 0 0; 0 1 0; 0 0 1]  BlockFunction=simmechanics.library.frames_transforms.rigid_transform
  Transform2 : sm_lib/Frames and Transforms/Rigid Transform  TranslationMethod=Cartesian  TranslationLengthUnit=mm  TranslationStandardAxis=+Z  TranslationStandardOffset=0  TranslationCartesianOffset=[0 0 360]  TranslationROffset=0  TranslationROffsetUnits=m  TranslationZOffset=0  TranslationZOffsetUnits=m  TranslationThetaOffset=0  TranslationThetaOffsetUnits=deg  RotationMethod=ArbitraryAxis  RotationAngleUnits=rad  RotationStandardAxis=+Z  RotationAngle=2.0943951023931953  RotationArbitraryAxis=[-0.57735026918962584 -0.57735026918962584 -0.57735026918962584]  FollAlignAxisA=+X  BaseAlignAxisA=+Y  FollAlignAxisB=+Y  BaseAlignAxisB=+Z  RotationMatrix=[1 0 0; 0 1 0; 0 0 1]  BlockFunction=simmechanics.library.frames_transforms.rigid_transform
  F : PMIOPort  Port=1  Side=Left
  F1 : PMIOPort  Port=2  Side=Right
  connections:
  Solid/RConn1 -- ReferenceFrame/RConn1 -- Transform2/LConn1 -- Transform/LConn1
  Transform/RConn1 -- F/RConn1
  Transform2/RConn1 -- F1/RConn1

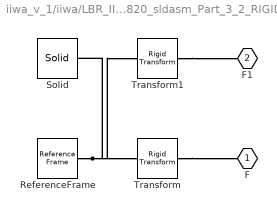
== system iiwa_v_1/iiwa/LBR_IIWA_14_R820_sldasm_Part_3_2_RIGID ==
  ReferenceFrame : sm_lib/Frames and Transforms/Reference Frame  BlockFunction=simmechanics.library.frames_transforms.reference_frame
  Solid : sm_lib/Body Elements/Solid  InertiaType=Custom  Mass=3.9510937025705992  MassUnits=kg  CenterOfMass=[-0.28186407311638517 41.985060717424616 418.80751382690903]  CenterOfMassUnits=mm  MomentsOfInertia=[30591.314957613846 30415.98862143857 11015.717417741856]  MomentsOfInertiaUnits=kg*mm^2  ProductsOfInertia=[4885.5830166425112 32.410847470181167 -21.913524538401049]  ProductsOfInertiaUnits=kg*mm^2  DensityBased=on  Density=1000  DensityUnits=kg/(m^3)  GraphicType=FromGeometry  MarkerShape=Sphere  MarkerSize=10  MarkerSizeUnits=m  GraphicVisPropType=SimpleVisualProperties  GraphicDiffuseColor=[1 0.40000000000000002 0]  GraphicSpecularColor=[0.5 0.5 0.5 1.0]  GraphicAmbientColor=[0.15 0.15 0.15 1.0]  GraphicEmissiveColor=[0.0 0.0 0.0 1.0]  GraphicShininess=75  GraphicOpacity=1  GeometryShape=FromFile  RectangleSize=[1 1]  RectangleSizeUnits=m  BrickDimensions=[1 1 1]  BrickDimensionUnits=m  CylinderRadius=1  CylinderRadiusUnits=m  CylinderLength=1  CylinderLengthUnits=m  SphereRadius=1  SphereRadiusUnits=m  EllipsoidRadii=[1 1 1]  EllipsoidRadiiUnits=m  ExtrusionCrossSection=[1 1; -1 1; -1 -1; 1 -1]  ExtrusionCrossSectionUnits=m  ExtrusionLength=1  ExtrusionLengthUnits=m  PolygonNumSides=3  PolygonOuterRadius=1  PolygonOuterRadiusUnits=m  ExtGeomFileType=STL  ExtGeomFileName=LBR IIWA 14 R820.sldasm-Part-3_Default_sldprt.STL  ExtGeomFileUnits=mm  RevolutionCrossSection=[1 1; 1 -1; 2 -1; 2 1]  RevolutionCrossSectionUnits=m  RevolutionExtent=Full  RevolutionAngle=180  RevolutionAngleUnits=deg  BlockFunction=simmechanics.library.body_elements.solid
  Transform : sm_lib/Frames and Transforms/Rigid Transform  TranslationMethod=Cartesian  TranslationLengthUnit=mm  TranslationStandardAxis=+Z  TranslationStandardOffset=0  TranslationCartesianOffset=[-0.43624370878124807 1.1013412404281553e-13 360.00000000000006]  TranslationROffset=0  TranslationROffsetUnits=m  TranslationZOffset=0  TranslationZOffsetUnits=m  TranslationThetaOffset=0  TranslationThetaOffsetUnits=deg  RotationMethod=ArbitraryAxis  RotationAngleUnits=rad  RotationStandardAxis=+Z  RotationAngle=2.0943951023931953  RotationArbitraryAxis=[-0.57735026918962584 -0.57735026918962584 -0.57735026918962584]  FollAlignAxisA=+X  BaseAlignAxisA=+Y  FollAlignAxisB=+Y  BaseAlignAxisB=+Z  RotationMatrix=[1 0 0; 0 1 0; 0 0 1]  BlockFunction=simmechanics.library.frames_transforms.rigid_transform
  Transform1 : sm_lib/Frames and Transforms/Rigid Transform  TranslationMethod=Cartesian  TranslationLengthUnit=mm  TranslationStandardAxis=+Z  TranslationStandardOffset=0  TranslationCartesianOffset=[-0.43624370878125873 1.1796119636642288e-13 564.5]  TranslationROffset=0  TranslationROffsetUnits=m  TranslationZOffset=0  TranslationZOffsetUnits=m  TranslationThetaOffset=0  TranslationThetaOffsetUnits=deg  RotationMethod=ArbitraryAxis  RotationAngleUnits=rad  RotationStandardAxis=+Z  RotationAngle=3.1415926535897931  RotationArbitraryAxis=[1 0 0]  FollAlignAxisA=+X  BaseAlignAxisA=+Y  FollAlignAxisB=+Y  BaseAlignAxisB=+Z  RotationMatrix=[1 0 0; 0 1 0; 0 0 1]  BlockFunction=simmechanics.library.frames_transforms.rigid_transform
  F : PMIOPort  Port=1  Side=Left
  F1 : PMIOPort  Port=2  Side=Right
  connections:
  Solid/RConn1 -- ReferenceFrame/RConn1 -- Transform/LConn1 -- Transform1/LConn1
  Transform/RConn1 -- F/RConn1
  Transform1/RConn1 -- F1/RConn1

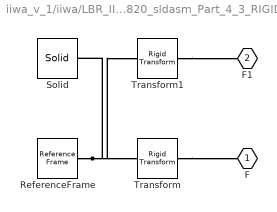
== system iiwa_v_1/iiwa/LBR_IIWA_14_R820_sldasm_Part_4_3_RIGID ==
  ReferenceFrame : sm_lib/Frames and Transforms/Reference Frame  BlockFunction=simmechanics.library.frames_transforms.reference_frame
  Solid : sm_lib/Body Elements/Solid  InertiaType=Custom  Mass=3.175233684000045  MassUnits=kg  CenterOfMass=[0.00045228460811316259 29.560619630803757 690.99757899972633]  CenterOfMassUnits=mm  MomentsOfInertia=[25080.930091979375 23809.456104382993 7608.5193786372311]  MomentsOfInertiaUnits=kg*mm^2  ProductsOfInertia=[-4873.7558441127658 -0.15707129067401196 -0.10518005394858314]  ProductsOfInertiaUnits=kg*mm^2  DensityBased=on  Density=1000  DensityUnits=kg/(m^3)  GraphicType=FromGeometry  MarkerShape=Sphere  MarkerSize=10  MarkerSizeUnits=m  GraphicVisPropType=SimpleVisualProperties  GraphicDiffuseColor=[1 0.40000000000000002 0]  GraphicSpecularColor=[0.5 0.5 0.5 1.0]  GraphicAmbientColor=[0.15 0.15 0.15 1.0]  GraphicEmissiveColor=[0.0 0.0 0.0 1.0]  GraphicShininess=75  GraphicOpacity=1  GeometryShape=FromFile  RectangleSize=[1 1]  RectangleSizeUnits=m  BrickDimensions=[1 1 1]  BrickDimensionUnits=m  CylinderRadius=1  CylinderRadiusUnits=m  CylinderLength=1  CylinderLengthUnits=m  SphereRadius=1  SphereRadiusUnits=m  EllipsoidRadii=[1 1 1]  EllipsoidRadiiUnits=m  ExtrusionCrossSection=[1 1; -1 1; -1 -1; 1 -1]  ExtrusionCrossSectionUnits=m  ExtrusionLength=1  ExtrusionLengthUnits=m  PolygonNumSides=3  PolygonOuterRadius=1  PolygonOuterRadiusUnits=m  ExtGeomFileType=STL  ExtGeomFileName=LBR IIWA 14 R820.sldasm-Part-4_Default_sldprt.STL  ExtGeomFileUnits=mm  RevolutionCrossSection=[1 1; 1 -1; 2 -1; 2 1]  RevolutionCrossSectionUnits=m  RevolutionExtent=Full  RevolutionAngle=180  RevolutionAngleUnits=deg  BlockFunction=simmechanics.library.body_elements.solid
  Transform : sm_lib/Frames and Transforms/Rigid Transform  TranslationMethod=Cartesian  TranslationLengthUnit=mm  TranslationStandardAxis=+Z  TranslationStandardOffset=0  TranslationCartesianOffset=[-1.4210854715202004e-14 0 564.5]  TranslationROffset=0  TranslationROffsetUnits=m  TranslationZOffset=0  TranslationZOffsetUnits=m  TranslationThetaOffset=0  TranslationThetaOffsetUnits=deg  RotationMethod=ArbitraryAxis  RotationAngleUnits=rad  RotationStandardAxis=+Z  RotationAngle=3.1415926535897931  RotationArbitraryAxis=[1 0 0]  FollAlignAxisA=+X  BaseAlignAxisA=+Y  FollAlignAxisB=+Y  BaseAlignAxisB=+Z  RotationMatrix=[1 0 0; 0 1 0; 0 0 1]  BlockFunction=simmechanics.library.frames_transforms.rigid_transform
  Transform1 : sm_lib/Frames and Transforms/Rigid Transform  TranslationMethod=Cartesian  TranslationLengthUnit=mm  TranslationStandardAxis=+Z  TranslationStandardOffset=0  TranslationCartesianOffset=[0 0.50000000000000044 780]  TranslationROffset=0  TranslationROffsetUnits=m  TranslationZOffset=0  TranslationZOffsetUnits=m  TranslationThetaOffset=0  TranslationThetaOffsetUnits=deg  RotationMethod=ArbitraryAxis  RotationAngleUnits=rad  RotationStandardAxis=+Z  RotationAngle=2.0943951023931953  RotationArbitraryAxis=[-0.57735026918962584 -0.57735026918962584 -0.57735026918962584]  FollAlignAxisA=+X  BaseAlignAxisA=+Y  FollAlignAxisB=+Y  BaseAlignAxisB=+Z  RotationMatrix=[1 0 0; 0 1 0; 0 0 1]  BlockFunction=simmechanics.library.frames_transforms.rigid_transform
  F : PMIOPort  Port=1  Side=Left
  F1 : PMIOPort  Port=2  Side=Right
  connections:
  Solid/RConn1 -- ReferenceFrame/RConn1 -- Transform/LConn1 -- Transform1/LConn1
  Transform/RConn1 -- F/RConn1
  Transform1/RConn1 -- F1/RConn1

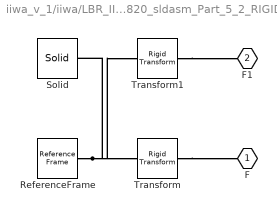
== system iiwa_v_1/iiwa/LBR_IIWA_14_R820_sldasm_Part_5_2_RIGID ==
  ReferenceFrame : sm_lib/Frames and Transforms/Reference Frame  BlockFunction=simmechanics.library.frames_transforms.reference_frame
  Solid : sm_lib/Body Elements/Solid  InertiaType=Custom  Mass=2.7391411686194478  MassUnits=kg  CenterOfMass=[0.0013008237739974492 -34.257165625619287 847.42501979348026]  CenterOfMassUnits=mm  MomentsOfInertia=[17201.112521940886 16394.587357464781 6135.8699139256114]  MomentsOfInertiaUnits=kg*mm^2  ProductsOfInertia=[-2845.2251083843989 -0.018768852953659411 -0.0031570610595521914]  ProductsOfInertiaUnits=kg*mm^2  DensityBased=on  Density=1000  DensityUnits=kg/(m^3)  GraphicType=FromGeometry  MarkerShape=Sphere  MarkerSize=10  MarkerSizeUnits=m  GraphicVisPropType=SimpleVisualProperties  GraphicDiffuseColor=[1 0.40000000000000002 0]  GraphicSpecularColor=[0.5 0.5 0.5 1.0]  GraphicAmbientColor=[0.15 0.15 0.15 1.0]  GraphicEmissiveColor=[0.0 0.0 0.0 1.0]  GraphicShininess=75  GraphicOpacity=1  GeometryShape=FromFile  RectangleSize=[1 1]  RectangleSizeUnits=m  BrickDimensions=[1 1 1]  BrickDimensionUnits=m  CylinderRadius=1  CylinderRadiusUnits=m  CylinderLength=1  CylinderLengthUnits=m  SphereRadius=1  SphereRadiusUnits=m  EllipsoidRadii=[1 1 1]  EllipsoidRadiiUnits=m  ExtrusionCrossSection=[1 1; -1 1; -1 -1; 1 -1]  ExtrusionCrossSectionUnits=m  ExtrusionLength=1  ExtrusionLengthUnits=m  PolygonNumSides=3  PolygonOuterRadius=1  PolygonOuterRadiusUnits=m  ExtGeomFileType=STL  ExtGeomFileName=LBR IIWA 14 R820.sldasm-Part-5_Default_sldprt.STL  ExtGeomFileUnits=mm  RevolutionCrossSection=[1 1; 1 -1; 2 -1; 2 1]  RevolutionCrossSectionUnits=m  RevolutionExtent=Full  RevolutionAngle=180  RevolutionAngleUnits=deg  BlockFunction=simmechanics.library.body_elements.solid
  Transform : sm_lib/Frames and Transforms/Rigid Transform  TranslationMethod=Cartesian  TranslationLengthUnit=mm  TranslationStandardAxis=+Z  TranslationStandardOffset=0  TranslationCartesianOffset=[-1.0658141036401503e-14 0.50000000000000711 779.99999999999989]  TranslationROffset=0  TranslationROffsetUnits=m  TranslationZOffset=0  TranslationZOffsetUnits=m  TranslationThetaOffset=0  TranslationThetaOffsetUnits=deg  RotationMethod=ArbitraryAxis  RotationAngleUnits=rad  RotationStandardAxis=+Z  RotationAngle=2.0943951023931953  RotationArbitraryAxis=[-0.57735026918962584 -0.57735026918962584 -0.57735026918962584]  FollAlignAxisA=+X  BaseAlignAxisA=+Y  FollAlignAxisB=+Y  BaseAlignAxisB=+Z  RotationMatrix=[1 0 0; 0 1 0; 0 0 1]  BlockFunction=simmechanics.library.frames_transforms.rigid_transform
  Transform1 : sm_lib/Frames and Transforms/Rigid Transform  TranslationMethod=Cartesian  TranslationLengthUnit=mm  TranslationStandardAxis=+Z  TranslationStandardOffset=0  TranslationCartesianOffset=[0 0 964]  TranslationROffset=0  TranslationROffsetUnits=m  TranslationZOffset=0  TranslationZOffsetUnits=m  TranslationThetaOffset=0  TranslationThetaOffsetUnits=deg  RotationMethod=ArbitraryAxis  RotationAngleUnits=rad  RotationStandardAxis=+Z  RotationAngle=3.1415926535897931  RotationArbitraryAxis=[1 0 0]  FollAlignAxisA=+X  BaseAlignAxisA=+Y  FollAlignAxisB=+Y  BaseAlignAxisB=+Z  RotationMatrix=[1 0 0; 0 1 0; 0 0 1]  BlockFunction=simmechanics.library.frames_transforms.rigid_transform
  F : PMIOPort  Port=1  Side=Left
  F1 : PMIOPort  Port=2  Side=Right
  connections:
  Solid/RConn1 -- ReferenceFrame/RConn1 -- Transform/LConn1 -- Transform1/LConn1
  Transform/RConn1 -- F/RConn1
  Transform1/RConn1 -- F1/RConn1

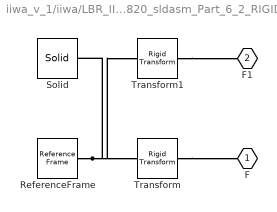
== system iiwa_v_1/iiwa/LBR_IIWA_14_R820_sldasm_Part_6_2_RIGID ==
  ReferenceFrame : sm_lib/Frames and Transforms/Reference Frame  BlockFunction=simmechanics.library.frames_transforms.reference_frame
  Solid : sm_lib/Body Elements/Solid  InertiaType=Custom  Mass=1.693757558760594  MassUnits=kg  CenterOfMass=[-0.12061181880451219 -21.387816054562705 1039.9701942770466]  CenterOfMassUnits=mm  MomentsOfInertia=[10080.087648851977 8702.6271828202862 4469.5074637142525]  MomentsOfInertiaUnits=kg*mm^2  ProductsOfInertia=[3090.3868314816905 -0.70385526974839641 1.5655850630883079]  ProductsOfInertiaUnits=kg*mm^2  DensityBased=on  Density=1000  DensityUnits=kg/(m^3)  GraphicType=FromGeometry  MarkerShape=Sphere  MarkerSize=10  MarkerSizeUnits=m  GraphicVisPropType=SimpleVisualProperties  GraphicDiffuseColor=[1 0.40000000000000002 0]  GraphicSpecularColor=[0.5 0.5 0.5 1.0]  GraphicAmbientColor=[0.15 0.15 0.15 1.0]  GraphicEmissiveColor=[0.0 0.0 0.0 1.0]  GraphicShininess=75  GraphicOpacity=1  GeometryShape=FromFile  RectangleSize=[1 1]  RectangleSizeUnits=m  BrickDimensions=[1 1 1]  BrickDimensionUnits=m  CylinderRadius=1  CylinderRadiusUnits=m  CylinderLength=1  CylinderLengthUnits=m  SphereRadius=1  SphereRadiusUnits=m  EllipsoidRadii=[1 1 1]  EllipsoidRadiiUnits=m  ExtrusionCrossSection=[1 1; -1 1; -1 -1; 1 -1]  ExtrusionCrossSectionUnits=m  ExtrusionLength=1  ExtrusionLengthUnits=m  PolygonNumSides=3  PolygonOuterRadius=1  PolygonOuterRadiusUnits=m  ExtGeomFileType=STL  ExtGeomFileName=LBR IIWA 14 R820.sldasm-Part-6_Default_sldprt.STL  ExtGeomFileUnits=mm  RevolutionCrossSection=[1 1; 1 -1; 2 -1; 2 1]  RevolutionCrossSectionUnits=m  RevolutionExtent=Full  RevolutionAngle=180  RevolutionAngleUnits=deg  BlockFunction=simmechanics.library.body_elements.solid
  Transform : sm_lib/Frames and Transforms/Rigid Transform  TranslationMethod=Cartesian  TranslationLengthUnit=mm  TranslationStandardAxis=+Z  TranslationStandardOffset=0  TranslationCartesianOffset=[7.1054273576010019e-15 3.5527136788005009e-15 963.99999999999989]  TranslationROffset=0  TranslationROffsetUnits=m  TranslationZOffset=0  TranslationZOffsetUnits=m  TranslationThetaOffset=0  TranslationThetaOffsetUnits=deg  RotationMethod=ArbitraryAxis  RotationAngleUnits=rad  RotationStandardAxis=+Z  RotationAngle=3.1415926535897931  RotationArbitraryAxis=[1 0 0]  FollAlignAxisA=+X  BaseAlignAxisA=+Y  FollAlignAxisB=+Y  BaseAlignAxisB=+Z  RotationMatrix=[1 0 0; 0 1 0; 0 0 1]  BlockFunction=simmechanics.library.frames_transforms.rigid_transform
  Transform1 : sm_lib/Frames and Transforms/Rigid Transform  TranslationMethod=Cartesian  TranslationLengthUnit=mm  TranslationStandardAxis=+Z  TranslationStandardOffset=0  TranslationCartesianOffset=[1.4155343563970746e-12 -60.700000000000003 1180]  TranslationROffset=0  TranslationROffsetUnits=m  TranslationZOffset=0  TranslationZOffsetUnits=m  TranslationThetaOffset=0  TranslationThetaOffsetUnits=deg  RotationMethod=ArbitraryAxis  RotationAngleUnits=rad  RotationStandardAxis=+Z  RotationAngle=2.0943951023931953  RotationArbitraryAxis=[0.57735026918962584 -0.57735026918962584 0.57735026918962584]  FollAlignAxisA=+X  BaseAlignAxisA=+Y  FollAlignAxisB=+Y  BaseAlignAxisB=+Z  RotationMatrix=[1 0 0; 0 1 0; 0 0 1]  BlockFunction=simmechanics.library.frames_transforms.rigid_transform
  F : PMIOPort  Port=1  Side=Left
  F1 : PMIOPort  Port=2  Side=Right
  connections:
  Solid/RConn1 -- ReferenceFrame/RConn1 -- Transform/LConn1 -- Transform1/LConn1
  Transform/RConn1 -- F/RConn1
  Transform1/RConn1 -- F1/RConn1

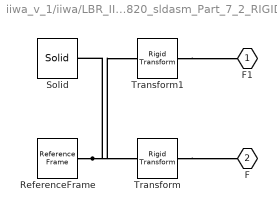
== system iiwa_v_1/iiwa/LBR_IIWA_14_R820_sldasm_Part_7_2_RIGID ==
  ReferenceFrame : sm_lib/Frames and Transforms/Reference Frame  BlockFunction=simmechanics.library.frames_transforms.reference_frame
  Solid : sm_lib/Body Elements/Solid  InertiaType=Custom  Mass=1.8086053219690341  MassUnits=kg  CenterOfMass=[0.0031143576123805862 0.34519354177310074 1180.5635303376107]  CenterOfMassUnits=mm  MomentsOfInertia=[4894.7919409782226 4685.8727117576109 3566.3042254280122]  MomentsOfInertiaUnits=kg*mm^2  ProductsOfInertia=[244.79413075305331 -0.04225590118291124 0.31482838300779464]  ProductsOfInertiaUnits=kg*mm^2  DensityBased=on  Density=1000  DensityUnits=kg/(m^3)  GraphicType=FromGeometry  MarkerShape=Sphere  MarkerSize=10  MarkerSizeUnits=m  GraphicVisPropType=SimpleVisualProperties  GraphicDiffuseColor=[1 0.40000000000000002 0]  GraphicSpecularColor=[0.5 0.5 0.5 1.0]  GraphicAmbientColor=[0.15 0.15 0.15 1.0]  GraphicEmissiveColor=[0.0 0.0 0.0 1.0]  GraphicShininess=75  GraphicOpacity=1  GeometryShape=FromFile  RectangleSize=[1 1]  RectangleSizeUnits=m  BrickDimensions=[1 1 1]  BrickDimensionUnits=m  CylinderRadius=1  CylinderRadiusUnits=m  CylinderLength=1  CylinderLengthUnits=m  SphereRadius=1  SphereRadiusUnits=m  EllipsoidRadii=[1 1 1]  EllipsoidRadiiUnits=m  ExtrusionCrossSection=[1 1; -1 1; -1 -1; 1 -1]  ExtrusionCrossSectionUnits=m  ExtrusionLength=1  ExtrusionLengthUnits=m  PolygonNumSides=3  PolygonOuterRadius=1  PolygonOuterRadiusUnits=m  ExtGeomFileType=STL  ExtGeomFileName=LBR IIWA 14 R820.sldasm-Part-7_Default_sldprt.STL  ExtGeomFileUnits=mm  RevolutionCrossSection=[1 1; 1 -1; 2 -1; 2 1]  RevolutionCrossSectionUnits=m  RevolutionExtent=Full  RevolutionAngle=180  RevolutionAngleUnits=deg  BlockFunction=simmechanics.library.body_elements.solid
  Transform : sm_lib/Frames and Transforms/Rigid Transform  TranslationMethod=Cartesian  TranslationLengthUnit=mm  TranslationStandardAxis=+Z  TranslationStandardOffset=0  TranslationCartesianOffset=[0 0 1260.3999999999999]  TranslationROffset=0  TranslationROffsetUnits=m  TranslationZOffset=0  TranslationZOffsetUnits=m  TranslationThetaOffset=0  TranslationThetaOffsetUnits=deg  RotationMethod=ArbitraryAxis  RotationAngleUnits=rad  RotationStandardAxis=+Z  RotationAngle=3.1415926535897931  RotationArbitraryAxis=[1 0 0]  FollAlignAxisA=+X  BaseAlignAxisA=+Y  FollAlignAxisB=+Y  BaseAlignAxisB=+Z  RotationMatrix=[1 0 0; 0 1 0; 0 0 1]  BlockFunction=simmechanics.library.frames_transforms.rigid_transform
  Transform1 : sm_lib/Frames and Transforms/Rigid Transform  TranslationMethod=Cartesian  TranslationLengthUnit=mm  TranslationStandardAxis=+Z  TranslationStandardOffset=0  TranslationCartesianOffset=[1.4210854715202004e-14 -60.699999999999989 1180]  TranslationROffset=0  TranslationROffsetUnits=m  TranslationZOffset=0  TranslationZOffsetUnits=m  TranslationThetaOffset=0  TranslationThetaOffsetUnits=deg  RotationMethod=ArbitraryAxis  RotationAngleUnits=rad  RotationStandardAxis=+Z  RotationAngle=2.0943951023931953  RotationArbitraryAxis=[0.57735026918962584 -0.57735026918962584 0.57735026918962584]  FollAlignAxisA=+X  BaseAlignAxisA=+Y  FollAlignAxisB=+Y  BaseAlignAxisB=+Z  RotationMatrix=[1 0 0; 0 1 0; 0 0 1]  BlockFunction=simmechanics.library.frames_transforms.rigid_transform
  F1 : PMIOPort  Port=1  Side=Left
  F : PMIOPort  Port=2  Side=Right
  connections:
  Solid/RConn1 -- ReferenceFrame/RConn1 -- Transform/LConn1 -- Transform1/LConn1
  Transform/RConn1 -- F/RConn1
  Transform1/RConn1 -- F1/RConn1

== matlab function iiwa_v_1/jacobian ==
  data: qDot1 output; q1 input; q2 input; q3 input; q4 input; q5 input; q6 input; q7 input; dx input; dy input; dz input; dA input; dB input; dC input; qDot2 output; qDot3 output; qDot4 output; qDot5 output; qDot6 output
function [qDot1,qDot2,qDot3,qDot4,qDot5,qDot6] = jacobian(q1,q2,q3,q4,q5,q6,q7,dx,dy,dz,dA,dB,dC)
%#codegen
Alpha = [0  -pi/2  pi/2 pi/2 -pi/2 -pi/2 pi/2] ;
a     = zeros(1,7) ;
d     = [.340 0 .400  0  .400 0 .141]; 
q     = [q1,q2,q3,q4,q5,q6,q7];
% q = deg2rad(q);
iiwa_DH_Table = [  Alpha'  a'     d'        q'];

T01 = Craig(iiwa_DH_Table(1,:));
T12 = Craig(iiwa_DH_Table(2,:));
T23 = Craig(iiwa_DH_Table(3,:));
T34 = Craig(iiwa_DH_Table(4,:));
T45 = Craig(iiwa_DH_Table(5,:));
T56 = Craig(iiwa_DH_Table(6,:));
T67 = Craig(iiwa_DH_Table(7,:));

    T02 =  T01 * T12;
    T03 =  T02 * T23;  
    T04 =  T03 * T34;  
    T05 =  T04 * T45;  
    T06 =  T05 * T56;  
    T07 =  T06 * T67;
    
z = [T01(1:3,3),T02(1:3,3),T03(1:3,3),T04(1:3,3),T05(1:3,3),T06(1:3,3),T07(1:3,3)];
    
Ojoint = [T01(1:3,4), T02(1:3,4), T03(1:3,4), T04(1:3,4), T05(1:3,4), T06(1:3,4), T07(1:3,4)];
Oend   = T07(1:3,4);
    
 j1 = [cross(z(:,1), Oend-Ojoint(:,1));z(:,1)];
 j2 = [cross(z(:,2), Oend-Ojoint(:,2));z(:,2)];
 j3 = [cross(z(:,3), Oend-Ojoint(:,3));z(:,3)];
 j4 = [cross(z(:,4), Oend-Ojoint(:,4));z(:,4)];
 j5 = [cross(z(:,5), Oend-Ojoint(:,5));z(:,5)];
 j6 = [cross(z(:,6), Oend-Ojoint(:,6));z(:,6)];
 j7 = [cross(z(:,7), Oend-Ojoint(:,7));z(:,7)];
    

%   jacobian7 = [j1 j2 j3 j4 j5 j6 j7]
  jacobian6 = [j1 j2 j4 j5 j6 j7];
%   pinv(jacobian7)*[0.2 0 0 0 0 0]'
 qDot =  inv(jacobian6)*[dx dy dz dA dB dC]';
 qDot1 = qDot(1);
 qDot2 = qDot(2);
 qDot3 = qDot(3);
 qDot4 = qDot(4);
 qDot5 = qDot(5);
 qDot6 = qDot(6);

== matlab function iiwa_v_1/FKin ==
  data: x output; q1 input; y output; q2 input; z output; q3 input; q4 input; q5 input; q6 input; q7 input; A output; B output; C output
function [x,y,z,A,B,C] = Fkin(q1,q2,q3,q4,q5,q6,q7)
%#codegen
Alpha = [0  -pi/2  pi/2 pi/2 -pi/2 -pi/2 pi/2] ;
a     = zeros(1,7) ;
d     = [.340 0 .400  0  .400 0 .141]; 
q     = [q1,q2,q3,q4,q5,q6,q7];
% q = deg2rad(q);
iiwa_DH_Table = [  Alpha'  a'     d'        q'];

T01 = Craig(iiwa_DH_Table(1,:));
T12 = Craig(iiwa_DH_Table(2,:));
T23 = Craig(iiwa_DH_Table(3,:));
T34 = Craig(iiwa_DH_Table(4,:));
T45 = Craig(iiwa_DH_Table(5,:));
T56 = Craig(iiwa_DH_Table(6,:));
T67 = Craig(iiwa_DH_Table(7,:));

    T02 =  T01 * T12;
    T03 =  T02 * T23;  
    T04 =  T03 * T34;  
    T05 =  T04 * T45;  
    T06 =  T05 * T56;  
    T07 =  T06 * T67;
    
R = T07(1:3,1:3);
% Rn = T07(1:3,1:3)*roty(-pi/2);    
Rn=R;
x = T07(1,4);
y = T07(2,4);
z = T07(3,4);
B = asin(Rn(1,3));
A = asin(-Rn(2,3)/cos(B));
C = asin(Rn(1,2)/-cos(B));
